simulink library "Library_SII_2018"  (R2018b)
settings: Solver=ode45  StartTime=0.0  StopTime=10.0  RelTol=1e-3  EnableMultiTasking=on
undefined symbols (not defined in the file or in its folder): coder, gcbh, r, simscape
libraries: fl_lib x157, nesl_utility x81, Library_SII2 x44, simulink x17, powerlib x12, mblibv1 x11, Simscape_SII_lib x11, elec_lib x10, Pneumatic_lib x4, $bdroot x2, peRmsMeasurement x1, powerlib_extras x1
(part 4 of 6)

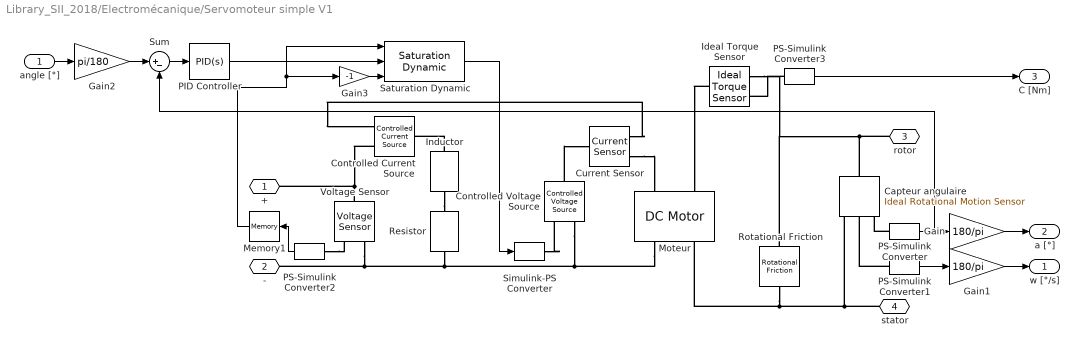
== system Library_SII_2018/Electromécanique/Servomoteur simple V1 ==
  angle [°] : Inport
  Capteur angulaire : fl_lib/Mechanical/Mechanical Sensors/Ideal Rotational Motion Sensor  offset=0 rad
  Controlled Current Source : fl_lib/Electrical/Electrical Sources/Controlled Current Source
  Controlled Voltage Source : fl_lib/Electrical/Electrical Sources/Controlled Voltage Source
  Current Sensor : fl_lib/Electrical/Electrical Sensors/Current Sensor
  Gain : Gain  Gain=180/pi
  Gain1 : Gain  Gain=180/pi
  Gain2 : Gain  Gain=pi/180
  Gain3 : Gain  Gain=-1
  Ideal Torque Sensor : fl_lib/Mechanical/Mechanical Sensors/Ideal Torque Sensor
  Inductor : fl_lib/Electrical/Electrical Elements/Inductor  l=L H  r=0 Ohm  g=1e-9 1/Ohm  i_specify=off  i_priority=High  i=0 A  i_nominal_specify=off  i_nominal_unit=A  i_nominal_value=1  v_specify=off  v_priority=High  v=0 V  v_nominal_specify=off  v_nominal_unit=V  v_nominal_value=1  i_L_specify=off  i_L_priority=High  i_L=0 A  i_L_nominal_specify=off  i_L_nominal_unit=A  i_L_nominal_value=1
  Memory1 : Memory  InheritSampleTime=on  LinearizeMemory=on
  Moteur : elec_lib/Actuators & Drivers/Rotational Actuators/DC Motor  parameterization=1  Ra=R Ohm  La=L H  emf_or_torque=1  Kv=K V/(rad/s)  Ki=6.876e-4 N*m/A  T_stall=2.4e-4 N*m  w_max=1.91e+4 rpm  w_rated=1.5e+4 rpm  P_rated=0.08 W  V_rated=1.5 V  J=0.001 kg*m^2  lam_param=1  lam=kv N*m/(rad/s)  i_noload=0 A  V_i_noload=1.5 V  speed0=0 rpm  alpha=0.00393 1/K  Tmeas=25 C  thermal_mass=100 J/K  initial_temperature=25 C
  PID Controller : simulink/Continuous/PID Controller  Controller=PID  Form=Parallel  TimeDomain=Continuous-time  SampleTime=-1  IntegratorMethod=Forward Euler  FilterMethod=Forward Euler  ControllerParametersSource=internal  P=P  I=I  D=D  UseFilter=on  N=100  TunerSelectOption=Transfer Function Based (PID Tuner App)  InitialConditionSource=internal  InitialConditionForIntegrator=0  InitialConditionForFilter=0  DifferentiatorICPrevScaledInput=0  ExternalReset=none  TrackingMode=off  Kt=1  LimitOutput=off  UpperSaturationLimit=inf  LowerSaturationLimit=-inf  LinearizeAsGain=on  AntiWindupMode=none  Kb=1  POutMin=[]  POutMax=[]  IOutMin=[]  IOutMax=[]  DOutMin=[]  DOutMax=[]  NOutMin=[]  NOutMax=[]  SumOutMin=[]  SumOutMax=[]  SaturationOutMin=[]  SaturationOutMax=[]  PParamMin=[]  PParamMax=[]  IParamMin=[]  IParamMax=[]  DParamMin=[]  DParamMax=[]  NParamMin=[]  NParamMax=[]  KbParamMin=[]  KbParamMax=[]  KtParamMin=[]  KtParamMax=[]  KbOutMin=[]  KbOutMax=[]  KtOutMin=[]  KtOutMax=[]  IntegratorOutMin=[]  IntegratorOutMax=[]  FilterOutMin=[]  FilterOutMax=[]  SumI1OutMin=[]  SumI1OutMax=[]  SumI2OutMin=[]  SumI2OutMax=[]  SumI3OutMin=[]  SumI3OutMax=[]  SumI4OutMin=[]  SumI4OutMax=[]  SumDOutMin=[]  SumDOutMax=[]  DifferentiatorOutMin=[]  DifferentiatorOutMax=[]  FilterDiffOutCoefMin=[]  FilterDiffOutCoefMax=[]  ReciprocalOutMin=[]  ReciprocalOutMax=[]  SumDenOutMin=[]  SumDenOutMax=[]  SumNumOutMin=[]  SumNumOutMax=[]  DivideOutMin=[]  DivideOutMax=[]  IntegratorContinuousStateAttributes=''  IntegratorStateMustResolveToSignalObject=off  IntegratorRTWStateStorageClass=Auto  FilterContinuousStateAttributes=''  FilterStateMustResolveToSignalObject=off  FilterRTWStateStorageClass=Auto  ParallelPVariant=InternalParameters  IdealPVariant=Disabled  IVariant=InternalParameters  DVariant=InternalParameters  IntegratorVariant=Continuous  SatVariant=Disabled  AWVariant=Passthrough  PCopyVariant=Disabled  TRVariant=Disabled  FdbkBlocksVariant=Forward  IdealPFdbkVariant=Disabled  SatFdbkVariant=Disabled  DerivativeFilterVariant=ContFilter  NVariant=InternalParameters  NCopyVariant=Disabled  FilterICVariant=InternalICsFilter  IntegratorICVariant=InternalICs  ExternalResetVariant=Disabled  TRSumVariant=Passthrough  SumFdbkVariant=Disabled  SumVariant=Sum_PID
  PS-Simulink Converter{,1..3} (4 alike) : nesl_utility/PS-Simulink Converter  PhysicalDomain=network_engine_domain  SubClassName=ps_output  LeftPortType=input  RightPortType=output  PseudoPeriodic=off  Frequencies=[]  Unit=1  AffineConversion=off
  Resistor : fl_lib/Electrical/Electrical Elements/Resistor  R=1/(1/R+1/R0) Ohm  i_specify=off  i_priority=High  i=0 A  i_nominal_specify=off  i_nominal_unit=A  i_nominal_value=1  v_specify=off  v_priority=High  v=0 V  v_nominal_specify=off  v_nominal_unit=V  v_nominal_value=1
  Rotational Friction : fl_lib/Mechanical/Rotational Elements/Rotational Friction  brkwy_trq=Cf*1.1 N*m  brkwy_vel=0.060623 rad/s  Col_trq=Cf N*m  visc_coef=0 N*m/(rad/s)  w_specify=off  w_priority=High  w=0 rad/s  w_nominal_specify=off  w_nominal_unit=rad/s  w_nominal_value=1  t_specify=off  t_priority=High  t=0 N*m  t_nominal_specify=off  t_nominal_unit=N*m  t_nominal_value=1
      settings: SourceProductName=Simscape
  Saturation Dynamic : simulink/Discontinuities/Saturation Dynamic  OutMin=[]  OutMax=[]  OutDataTypeStr=Inherit: Same as second input  OutDataType=fixdt(1, 16)  OutScaling=2^-10  DoSatur=off
  Simulink-PS Converter : nesl_utility/Simulink-PS Converter  PhysicalDomain=network_engine_domain  SubClassName=ps_input  LeftPortType=input  RightPortType=output  PseudoPeriodic=off  Frequencies=[]  NoiseDistribution=none  NoiseParameters=[]  Unit=1  AffineConversion=off  FilteringAndDerivatives=zero  SimscapeFilterOrder=1  InputFilterTimeConstant=0.001  UdotUserProvided=1
  Sum : Sum  Inputs=|+-
  Voltage Sensor : fl_lib/Electrical/Electrical Sensors/Voltage Sensor
  + : PMIOPort  Side=Left
  - : PMIOPort  Port=2  Side=Left
  rotor : PMIOPort  Port=3  Side=Right
  stator : PMIOPort  Port=4  Side=Right
  w [°/s] : Outport
  a [°] : Outport  Port=2
  C [Nm] : Outport  Port=3
  wires:
  PS-Simulink Converter3/1 -> C [Nm]/1
  PS-Simulink Converter1/1 -> Gain1/1
  Sum/1 -> PID Controller/1
  angle [°]/1 -> Gain2/1
  Gain/1 -> a [°]/1
  Gain1/1 -> w [°/s]/1
  Gain2/1 -> Sum/1
  PID Controller/1 -> Saturation Dynamic/2
  Saturation Dynamic/1 -> Simulink-PS Converter/1
  Gain3/1 -> Saturation Dynamic/3
  Memory1/1 -> Saturation Dynamic/1, Gain3/1
  PS-Simulink Converter/1 -> Sum/2, Gain/1
  PS-Simulink Converter2/1 -> Memory1/1
  connections:
  PS-Simulink Converter3/LConn1 -- Ideal Torque Sensor/RConn2
  Ideal Torque Sensor/LConn1 -- Moteur/LConn2
  stator/RConn1 -- Rotational Friction/RConn1 -- Moteur/RConn2 -- Capteur angulaire/RConn1
  PS-Simulink Converter1/LConn1 -- Capteur angulaire/RConn2
  PS-Simulink Converter/LConn1 -- Capteur angulaire/RConn3
  Capteur angulaire/LConn1 -- Rotational Friction/LConn1 -- Ideal Torque Sensor/RConn1 -- rotor/RConn1
  Moteur/RConn1 -- Controlled Voltage Source/RConn2 -- Resistor/RConn1 -- -/RConn1 -- Voltage Sensor/RConn2
  Controlled Voltage Source/LConn1 -- Current Sensor/LConn1
  Controlled Current Source/RConn2 -- Voltage Sensor/LConn1 -- +/RConn1
  Simulink-PS Converter/RConn1 -- Controlled Voltage Source/RConn1
  Current Sensor/RConn2 -- Moteur/LConn1
  Current Sensor/RConn1 -- Controlled Current Source/RConn1
  PS-Simulink Converter2/LConn1 -- Voltage Sensor/RConn1
  Inductor/LConn1 -- Controlled Current Source/LConn1
  Inductor/RConn1 -- Resistor/LConn1

== system Library_SII_2018/Electronique/Ampèremètre ==
  Current Sensor : fl_lib/Electrical/Electrical Sensors/Current Sensor
  S-PS : nesl_utility/PS-Simulink Converter  PhysicalDomain=network_engine_domain  SubClassName=ps_output  LeftPortType=input  RightPortType=output  PseudoPeriodic=off  Frequencies=[]  Unit=A  AffineConversion=off
  Conn1 : PMIOPort  Side=Left
  Conn2 : PMIOPort  Port=2  Side=Right
  Out1 : Outport
  wires:
  S-PS/1 -> Out1/1
  connections:
  Current Sensor/RConn1 -- S-PS/LConn1
  Conn2/RConn1 -- Current Sensor/RConn2
  Conn1/RConn1 -- Current Sensor/LConn1

== system Library_SII_2018/Electronique/Bobine entrée ==
  Electromagnetic Converter : fl_lib/Magnetic/Magnetic Elements/Electromagnetic Converter  Nw=N  i_specify=off  i_priority=None  i=0 A  i_nominal_specify=off  i_nominal_unit=A  i_nominal_value=1  v_specify=off  v_priority=None  v=0 V  v_nominal_specify=off  v_nominal_unit=V  v_nominal_value=1  mmf_specify=off  mmf_priority=None  mmf=0 A  mmf_nominal_specify=off  mmf_nominal_unit=A  mmf_nominal_value=1  phi_specify=off  phi_priority=High  phi=0 Wb  phi_nominal_specify=off  phi_nominal_unit=Wb  phi_nominal_value=1
      settings: SourceProductName=Simscape  SourceProductBaseCode=SS
  Fundamental Reluctance : fl_lib/Magnetic/Magnetic Elements/Fundamental Reluctance  R=4*l/(mu0*pi*D^2) 1/H  phi_specify=off  phi_priority=None  phi=0 Wb  phi_nominal_specify=off  phi_nominal_unit=Wb  phi_nominal_value=1  mmf_specify=off  mmf_priority=None  mmf=0 A  mmf_nominal_specify=off  mmf_nominal_unit=A  mmf_nominal_value=1
      settings: SourceProductName=Simscape  SourceProductBaseCode=SS
  Inductor : fl_lib/Electrical/Electrical Elements/Inductor  l=mu0*pi*D^2/4*N^2/l H  r=0 Ohm  g=1e-20 1/Ohm  i_specify=off  i_priority=None  i=0 A  i_nominal_specify=off  i_nominal_unit=A  i_nominal_value=1  v_specify=off  v_priority=None  v=0 V  v_nominal_specify=off  v_nominal_unit=V  v_nominal_value=1  i_L_specify=off  i_L_priority=High  i_L=0 A  i_L_nominal_specify=off  i_L_nominal_unit=A  i_L_nominal_value=1
  Resistor : fl_lib/Electrical/Electrical Elements/Resistor  R=rho*pi*D*N/s Ohm  i_specify=off  i_priority=None  i=0 A  i_nominal_specify=off  i_nominal_unit=A  i_nominal_value=1  v_specify=off  v_priority=None  v=0 V  v_nominal_specify=off  v_nominal_unit=V  v_nominal_value=1
  + : PMIOPort  Side=Left
  - : PMIOPort  Port=2  Side=Left
  N : PMIOPort  Port=3  Side=Right
  S : PMIOPort  Port=4  Side=Right
  connections:
  -/RConn1 -- Inductor/LConn1
  +/RConn1 -- Resistor/LConn1
  Inductor/RConn1 -- Electromagnetic Converter/LConn2
  Fundamental Reluctance/RConn1 -- S/RConn1 -- Electromagnetic Converter/RConn2
  Resistor/RConn1 -- Electromagnetic Converter/LConn1
  Electromagnetic Converter/RConn1 -- Fundamental Reluctance/LConn1 -- N/RConn1

== system Library_SII_2018/Electronique/Cellule Photovoltaique SPS ==
  Ta : Inport
  Ir : Inport  Port=2
  Add : Sum  Inputs=-+
  Courant de saturation diode : Subsystem
  Courant diode : Subsystem
  Courant gégéré par l'éclairement : Subsystem
  Estimation température cellule : Subsystem
  Fcn : Fcn  Expr=u(1)+beta*(u(2)-Tjref)
  Is : powerlib/Electrical Sources/Controlled Current Source  Initialize=on  Source_Type=AC  Amplitude=0  Phase=0  Frequency=0  Measurements=None
      settings: SourceProductName=Simscape Electrical
  Mux : Mux  Inputs=2
  Rs : powerlib/Elements/Series RLC Branch  LConnTagsString=__new0  RConnTagsString=__new0  BranchType=R  Resistance=Rs  Inductance=1e-3  SetiL0=off  InitialCurrent=0  Capacitance=1e-6  Setx0=off  InitialVoltage=0  Measurements=None
      settings: SourceProductName=Simscape Electrical
  Rsh : powerlib/Elements/Series RLC Branch  LConnTagsString=__new0  RConnTagsString=__new0  BranchType=R  Resistance=Rsh  Inductance=1e-3  SetiL0=off  InitialCurrent=0  Capacitance=1e-6  Setx0=off  InitialVoltage=0  Measurements=None
      settings: SourceProductName=Simscape Electrical
  Température optimale (constructeur) : Constant  Value=45
  Tension thermique : Subsystem
  Transport Delay : TransportDelay  DelayTime=0.001
  V : powerlib/Measurements/Voltage Measurement  PhasorSimulation=off  OutputType=Complex  PSBequivalent=0
      settings: SourceProductName=Simscape Electrical
  + : PMIOPort  Tag=PMCPort  Side=Right
  - : PMIOPort  Tag=PMCPort  Port=2  Side=Right
  wires:
  Add/1 -> Is/1
  Estimation température cellule/1(Tj) -> Courant gégéré par l'éclairement/1(Tj), Tension thermique/1(Tj (°C)), Courant de saturation diode/1(Tj)
  Température optimale (constructeur)/1 -> Estimation température cellule/1(noct)
  Ta/1 -> Estimation température cellule/2(Ta)
  Ir/1 -> Estimation température cellule/3(Ir), Courant gégéré par l'éclairement/2(Ir)
  Courant gégéré par l'éclairement/1(Iph) -> Add/2
  Courant diode/1(Id) -> Add/1
  Mux/1 -> Fcn/1
  V/1 -> Courant diode/1(Vd)
  Tension thermique/1(Vt (V)) -> Courant diode/3(Vt), Courant de saturation diode/2(Vt)
  Courant de saturation diode/1(Id0) -> Courant diode/2(I0d)
  connections:
  V/LConn2 -- -/RConn1 -- Is/LConn1 -- Rsh/RConn1
  Is/RConn1 -- Rs/LConn1 -- V/LConn1 -- Rsh/LConn1
  Rs/RConn1 -- +/RConn1

== system Library_SII_2018/Electronique/Cellule Photovoltaique avec capteurs U et I SimElectronics ==
  Ir : Inport
  Constant : Constant  Value=shunt
  Current Sensor : fl_lib/Electrical/Electrical Sensors/Current Sensor
  PS-Simulink Converter : nesl_utility/PS-Simulink Converter  PhysicalDomain=network_engine_domain  SubClassName=ps_output  LeftPortType=input  RightPortType=output  PseudoPeriodic=off  Frequencies=[]  Unit=1  AffineConversion=off
  PS-Simulink Converter1 : nesl_utility/PS-Simulink Converter  PhysicalDomain=network_engine_domain  SubClassName=ps_output  LeftPortType=input  RightPortType=output  PseudoPeriodic=off  Frequencies=[]  Unit=1  AffineConversion=off
  Simulink-PS Converter : nesl_utility/Simulink-PS Converter  PhysicalDomain=network_engine_domain  SubClassName=ps_input  LeftPortType=input  RightPortType=output  PseudoPeriodic=off  Frequencies=[]  NoiseDistribution=none  NoiseParameters=[]  Unit=1  AffineConversion=off  FilteringAndDerivatives=zero  SimscapeFilterOrder=1  InputFilterTimeConstant=.001  UdotUserProvided=0
  Simulink-PS Converter1 : nesl_utility/Simulink-PS Converter  PhysicalDomain=network_engine_domain  SubClassName=ps_input  LeftPortType=input  RightPortType=output  PseudoPeriodic=off  Frequencies=[]  NoiseDistribution=none  NoiseParameters=[]  Unit=1  AffineConversion=off  FilteringAndDerivatives=zero  SimscapeFilterOrder=1  InputFilterTimeConstant=.001  UdotUserProvided=0
  Solar Cell : elec_lib/Sources/Solar Cell  prm=1  Isc=Icc A  Voc=Vco V  Is=1e-6 A  Is2=0 A  Iph=7.34 A  Ir0=IRef W/m^2  ec=Qf  N2=2  Rs=0 Ohm  Rp=Inf Ohm  N_series=1  TIPH1=0 1/K  EG=1.11 eV  TXIS1=3  TXIS2=3  TRS1=0  TRP1=0  Tmeas=TRef C  TFIXED=Tcell C  thermal_mass=100 J/K  initial_temperature=25 C
      settings: SourceProductName=Simscape Electronics  SourceProductBaseCode=SN
  Switch : fl_lib/Electrical/Electrical Elements/Switch  R_closed=1e-8 Ohm  G_open=1e-8 1/Ohm  Threshold=0  i_specify=off  i_priority=High  i=0 A  i_nominal_specify=off  i_nominal_unit=A  i_nominal_value=1  v_specify=off  v_priority=High  v=0 V  v_nominal_specify=off  v_nominal_unit=V  v_nominal_value=1
      settings: SourceProductName=Simscape
  Voltage Sensor : fl_lib/Electrical/Electrical Sensors/Voltage Sensor
  + : PMIOPort  Side=Right
  - : PMIOPort  Port=2  Side=Right
  I : Outport
  U : Outport  Port=2
  wires:
  Ir/1 -> Simulink-PS Converter1/1
  PS-Simulink Converter/1 -> I/1
  PS-Simulink Converter1/1 -> U/1
  Constant/1 -> Simulink-PS Converter/1
  connections:
  Simulink-PS Converter1/RConn1 -- Solar Cell/LConn1
  Switch/RConn2 -- Voltage Sensor/RConn2 -- -/RConn1 -- Solar Cell/RConn1
  Voltage Sensor/LConn1 -- Current Sensor/RConn2 -- +/RConn1
  Voltage Sensor/RConn1 -- PS-Simulink Converter1/LConn1
  Current Sensor/RConn1 -- PS-Simulink Converter/LConn1
  Switch/LConn1 -- Current Sensor/LConn1 -- Solar Cell/LConn2
  Simulink-PS Converter/RConn1 -- Switch/RConn1

== system Library_SII_2018/Electronique/Diode ==
  Tj (°C) : Inport
  Courant de saturation diode : Subsystem
  Courant diode : Subsystem
  Is : powerlib/Electrical Sources/Controlled Current Source  Initialize=on  Source_Type=AC  Amplitude=0  Phase=0  Frequency=0  Measurements=None
      settings: SourceProductName=Simscape Electrical
  Tension thermique : Subsystem
  V : powerlib/Measurements/Voltage Measurement  PhasorSimulation=off  OutputType=Complex  PSBequivalent=0
      settings: SourceProductName=Simscape Electrical
  C : PMIOPort  Tag=PMCPort  Side=Right
  A : PMIOPort  Tag=PMCPort  Port=2  Side=Left
  wires:
  Courant diode/1(Id) -> Is/1
  V/1 -> Courant diode/1(Vd)
  Courant de saturation diode/1(Id0) -> Courant diode/2(I0d)
  Tj (°C)/1 -> Courant de saturation diode/1(Tj), Tension thermique/1(Tj (°C))
  Tension thermique/1(Vt) -> Courant diode/3(Vt)
  connections:
  Is/LConn1 -- C/RConn1 -- V/LConn2
  Is/RConn1 -- A/RConn1 -- V/LConn1

== system Library_SII_2018/Electronique/Hacheur (PWM) ==
  Consigne (0 --> 100) : Inport
  Controlled Voltage Source1 : fl_lib/Electrical/Electrical Sources/Controlled Voltage Source
  Gain1 : Gain  Gain=A  OutDataTypeStr=double
  Relational Operator : RelationalOperator  RndMeth=Nearest
  Repeating Sequence : simulink/Sources/Repeating Sequence  rep_seq_t=[0 1/f]  rep_seq_y=[0 100]
  Simulink-PS Converter : nesl_utility/Simulink-PS Converter  PhysicalDomain=network_engine_domain  SubClassName=ps_input  LeftPortType=input  RightPortType=output  PseudoPeriodic=off  Frequencies=[]  NoiseDistribution=none  NoiseParameters=[]  Unit=1  AffineConversion=off  FilteringAndDerivatives=zero  SimscapeFilterOrder=1  InputFilterTimeConstant=0.001  UdotUserProvided=1
  + : PMIOPort  Side=Right
  - : PMIOPort  Port=2  Side=Right
  Tension : Outport
  wires:
  Relational Operator/1 -> Gain1/1
  Gain1/1 -> Tension/1, Simulink-PS Converter/1
  Consigne (0 --> 100)/1 -> Relational Operator/1
  Repeating Sequence/1 -> Relational Operator/2
  connections:
  Controlled Voltage Source1/RConn1 -- Simulink-PS Converter/RConn1
  -/RConn1 -- Controlled Voltage Source1/RConn2
  +/RConn1 -- Controlled Voltage Source1/LConn1

== system Library_SII_2018/Electronique/Hacheur (PWM) Tension variable ==
  Consigne (0 --> 100) : Inport
  Tension [V] : Inport  Port=2
  Controlled Voltage Source1 : fl_lib/Electrical/Electrical Sources/Controlled Voltage Source
  Product : Product
  Relational Operator : RelationalOperator  RndMeth=Nearest
  Repeating Sequence : simulink/Sources/Repeating Sequence  rep_seq_t=[0 1/f]  rep_seq_y=[0 100]
  Simulink-PS Converter : nesl_utility/Simulink-PS Converter  PhysicalDomain=network_engine_domain  SubClassName=ps_input  LeftPortType=input  RightPortType=output  PseudoPeriodic=off  Frequencies=[]  NoiseDistribution=none  NoiseParameters=[]  Unit=1  AffineConversion=off  FilteringAndDerivatives=zero  SimscapeFilterOrder=1  InputFilterTimeConstant=0.001  UdotUserProvided=1
  + : PMIOPort  Side=Right
  - : PMIOPort  Port=2  Side=Right
  Tension : Outport
  wires:
  Repeating Sequence/1 -> Relational Operator/2
  Consigne (0 --> 100)/1 -> Relational Operator/1
  Product/1 -> Simulink-PS Converter/1, Tension/1
  Relational Operator/1 -> Product/2
  Tension [V]/1 -> Product/1
  connections:
  +/RConn1 -- Controlled Voltage Source1/LConn1
  -/RConn1 -- Controlled Voltage Source1/RConn2
  Controlled Voltage Source1/RConn1 -- Simulink-PS Converter/RConn1

== system Library_SII_2018/Electronique/Interrupteur ==
  In1 : Inport
  S-PS1 : nesl_utility/Simulink-PS Converter  PhysicalDomain=network_engine_domain  SubClassName=ps_input  LeftPortType=input  RightPortType=output  PseudoPeriodic=off  Frequencies=[]  NoiseDistribution=none  NoiseParameters=[]  Unit=1  AffineConversion=off  FilteringAndDerivatives=zero  SimscapeFilterOrder=1  InputFilterTimeConstant=.001  UdotUserProvided=0
  Switch : fl_lib/Electrical/Electrical Elements/Switch  R_closed=1e-8 Ohm  G_open=1e-8 1/Ohm  Threshold=0  i_specify=off  i_priority=High  i=0 A  i_nominal_specify=off  i_nominal_unit=A  i_nominal_value=1  v_specify=off  v_priority=High  v=0 V  v_nominal_specify=off  v_nominal_unit=V  v_nominal_value=1
      settings: SourceProductName=Simscape
  Conn1 : PMIOPort  Side=Left
  Conn2 : PMIOPort  Port=2  Side=Right
  wires:
  In1/1 -> S-PS1/1
  connections:
  S-PS1/RConn1 -- Switch/RConn1
  Conn1/RConn1 -- Switch/LConn1
  Conn2/RConn1 -- Switch/RConn2

== system Library_SII_2018/Electronique/Mesure Puissance RMS ==
  Amperemetre : $bdroot/Electronique/Ampèremètre
  Mux : Mux  Inputs=3
  Product : Product
  RMS Measurement : peRmsMeasurement/RMS Measurement  LabelModeActiveChoice=Total  F=ff  SpecifyHarmonics=off  K=[0 1 2]  Ts=0
  Voltmetre : $bdroot/Electronique/Voltmètre
  E : PMIOPort  Side=Left
  Ref : PMIOPort  Port=2  Side=Left
  S : PMIOPort  Port=3  Side=Right
  "[I, U, P]" : Outport
  wires:
  Mux/1 -> RMS Measurement/1
  RMS Measurement/1 -> "[I, U, P]"/1
  Product/1 -> Mux/3  "Puissance"
  Voltmetre/1 -> Product/2, Mux/2  "Upv"
  Amperemetre/1 -> Product/1, Mux/1  "Ipv"
  connections:
  Amperemetre/RConn1 -- S/RConn1 -- Voltmetre/LConn1
  Voltmetre/RConn1 -- Ref/RConn1
  Amperemetre/LConn1 -- E/RConn1

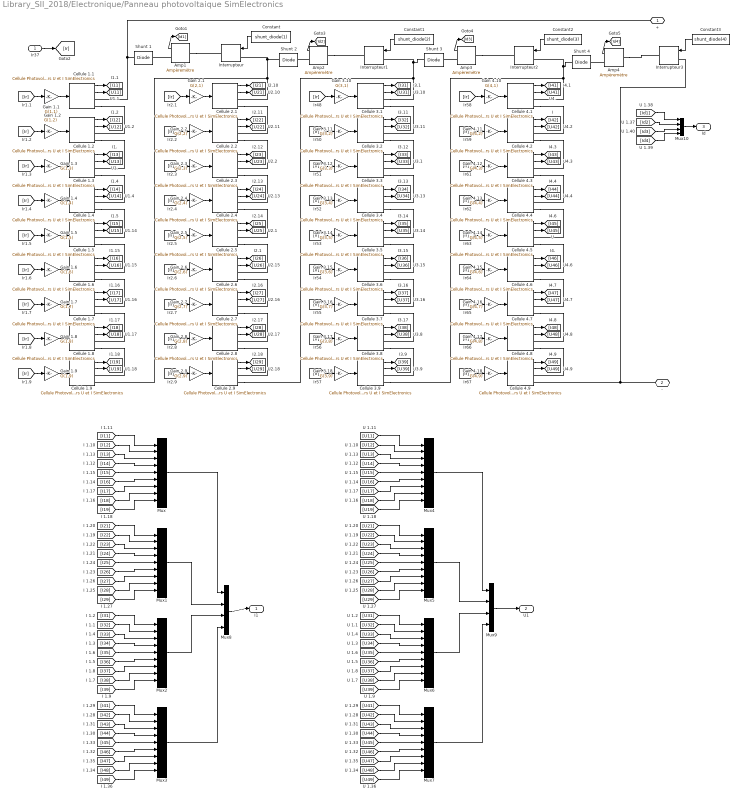
== system Library_SII_2018/Electronique/Panneau photovoltaique SimElectronics ==
  Ir37 : Inport
  Amp{1..4} (4 alike) : Library_SII2/Electronique/Ampèremètre
  Cellule 1.1 : Library_SII2/Electronique/Cellule Photovoltaique avec capteurs U et I SimElectronics  typcell=polycristallin  Icc=Icc  Vco=Vco  Tcell=Tcell  shunt=0  mesure=off  IRef=1000  TRef=25  Qf=1.4
  Cellule 1.{2..8} (7 alike) : Library_SII2/Electronique/Cellule Photovoltaique avec capteurs U et I SimElectronics  typcell=polycristallin  Icc=Icc  Vco=Vco  Tcell=Tcell  shunt=0  mesure=off  IRef=1000  TRef=25  Qf=1.5
  Cellule 1.9 : Library_SII2/Electronique/Cellule Photovoltaique avec capteurs U et I SimElectronics  typcell=polycristallin  Icc=Icc  Vco=Vco  Tcell=Tcell  shunt=1  mesure=off  IRef=1000  TRef=25  Qf=1.5
  Cellule 2.{1..7} (7 alike) : Library_SII2/Electronique/Cellule Photovoltaique avec capteurs U et I SimElectronics  typcell=polycristallin  Icc=Icc  Vco=Vco  Tcell=Tcell  shunt=0  mesure=off  IRef=1000  TRef=25  Qf=1.5
  Cellule 2.8 : Library_SII2/Electronique/Cellule Photovoltaique avec capteurs U et I SimElectronics  typcell=polycristallin  Icc=Icc  Vco=Vco  Tcell=Tcell  shunt=0  mesure=off  IRef=1000  TRef=25  Qf=10
  Cellule 2.9 : Library_SII2/Electronique/Cellule Photovoltaique avec capteurs U et I SimElectronics  typcell=polycristallin  Icc=Icc  Vco=Vco  Tcell=Tcell  shunt=1  mesure=off  IRef=1000  TRef=25  Qf=1.5
  Cellule 3.{1..8} (8 alike) : Library_SII2/Electronique/Cellule Photovoltaique avec capteurs U et I SimElectronics  typcell=polycristallin  Icc=Icc  Vco=Vco  Tcell=Tcell  shunt=0  mesure=off  IRef=1000  TRef=25  Qf=1.5
  Cellule 3.9 : Library_SII2/Electronique/Cellule Photovoltaique avec capteurs U et I SimElectronics  typcell=polycristallin  Icc=Icc  Vco=Vco  Tcell=Tcell  shunt=1  mesure=off  IRef=1000  TRef=25  Qf=1.5
  Cellule 4.{1..8} (8 alike) : Library_SII2/Electronique/Cellule Photovoltaique avec capteurs U et I SimElectronics  typcell=polycristallin  Icc=Icc  Vco=Vco  Tcell=Tcell  shunt=0  mesure=off  IRef=1000  TRef=25  Qf=1.5
  Cellule 4.9 : Library_SII2/Electronique/Cellule Photovoltaique avec capteurs U et I SimElectronics  typcell=polycristallin  Icc=Icc  Vco=Vco  Tcell=Tcell  shunt=1  mesure=off  IRef=1000  TRef=25  Qf=1.5
  Constant : Constant  Value=shunt_diode(1)
  Constant1 : Constant  Value=shunt_diode(2)
  Constant2 : Constant  Value=shunt_diode(3)
  Constant3 : Constant  Value=shunt_diode(4)
  Gain 1.1 : Gain  Gain=G(1,1)
  Gain 1.2 : Gain  Gain=G(1,2)
  Gain 1.3 : Gain  Gain=G(1,3)
  Gain 1.4 : Gain  Gain=G(1,4)
  Gain 1.5 : Gain  Gain=G(1,5)
  Gain 1.6 : Gain  Gain=G(1,6)
  Gain 1.7 : Gain  Gain=G(1,7)
  Gain 1.8 : Gain  Gain=G(1,8)
  Gain 1.9 : Gain  Gain=G(1,9)
  Gain 2.1 : Gain  Gain=G(2,1)
  Gain 2.2 : Gain  Gain=G(2,2)
  Gain 2.3 : Gain  Gain=G(2,3)
  Gain 2.4 : Gain  Gain=G(2,4)
  Gain 2.5 : Gain  Gain=G(2,5)
  Gain 2.6 : Gain  Gain=G(2,6)
  Gain 2.7 : Gain  Gain=G(2,7)
  Gain 2.8 : Gain  Gain=G(2,8)
  Gain 2.9 : Gain  Gain=G(2,9)
  Gain 3.10 : Gain  Gain=G(3,1)
  Gain 3.11 : Gain  Gain=G(3,2)
  Gain 3.12 : Gain  Gain=G(3,3)
  Gain 3.13 : Gain  Gain=G(3,4)
  Gain 3.14 : Gain  Gain=G(3,5)
  Gain 3.15 : Gain  Gain=G(3,6)
  Gain 3.16 : Gain  Gain=G(3,7)
  Gain 3.17 : Gain  Gain=G(3,8)
  Gain 3.18 : Gain  Gain=G(3,9)
  Gain 4.10 : Gain  Gain=G(4,1)
  Gain 4.11 : Gain  Gain=G(4,2)
  Gain 4.12 : Gain  Gain=G(4,3)
  Gain 4.13 : Gain  Gain=G(4,4)
  Gain 4.14 : Gain  Gain=G(4,5)
  Gain 4.15 : Gain  Gain=G(4,6)
  Gain 4.16 : Gain  Gain=G(4,7)
  Gain 4.17 : Gain  Gain=G(4,8)
  Gain 4.18 : Gain  Gain=G(4,9)
  Interrupteur{,1..3} (4 alike) : Library_SII2/Electronique/Interrupteur
  Mux{,1..7} (8 alike) : Mux  Inputs=9
  Mux10 : Mux
  Mux8 : Mux
  Mux9 : Mux
  Shunt {1..4} (4 alike) : elec_lib/Semiconductor Devices/Diode  ModelType=1  Vf=0.6 V  Ron=0.3 Ohm  Goff=1e-8 S  Rz=0.3 Ohm  Vz=50 V  C_PWL=5 pF  prmExp=1  I12=[ 0.0137 0.545 ] A  V12=[ 0.6 0.7 ] V  I1=0.0137 A  V1=0.6 V  IS=1e-12 A  ec=1  RS=0.01 Ohm  Tmeas=25 C  BV=Inf V  C_param=1  CJ0=5 pF  VJ=1 V  Mgrad=0.5  Vvec=[ 0.1 10 100 ] V  Cvec=[ 3.5 1 0.4 ] pF  FC=0.5  Q_param=1  Irrm=-7.15 A  iF=4 A  didt=-750 A/us  trr=115 ns  TT=50 ns  tau=100 ns  T_param=1  IS_T2=1.25e-7 A  I1_T2=0.245 A  V1_T2=0.5 V  Tmeas2=125 C  EG_param=1  EG=1.11 eV  XTI_param=1  XTI=3  dBVdT=0 V/K  Tdevice=25 C  i_capacitor_specify=off  i_capacitor_priority=High  i_capacitor=0 A  i_capacitor_nominal_specify=off  i_capacitor_nominal_unit=A  i_capacitor_nominal_value=1  v_capacitor_specify=off  v_capacitor_priority=None  v_capacitor=0 V  v_capacitor_nominal_specify=off  v_capacitor_nominal_unit=V  v_capacitor_nominal_value=1  Rth=[ 0 10 ] K/W  thermal_mass_parameterization=1  thermal_mass=[ 0 1 ] J/K  thermal_time_constant=[ 0 10 ] s  thermal_mass_initial_temperatures=[ 25 25 ] C
      settings: SourceProductName=Simscape Electronics  SourceProductBaseCode=SN
  + : PMIOPort  Side=Right
  - : PMIOPort  Port=2  Side=Right
  I1 : Outport
  U1 : Outport  Port=2
  Id : Outport  Port=3
  wires:
  Ir37/1 -> [Ir]
  [Ir] -> Gain 1.1/1
  Gain 1.1/1 -> Cellule 1.1/1
  Cellule 1.1/1 -> [I11]
  Cellule 1.1/2 -> [U11]
  [Ir] -> Gain 1.2/1
  Gain 1.2/1 -> Cellule 1.2/1
  Cellule 1.2/1 -> [I12]
  Cellule 1.2/2 -> [U12]
  [Ir] -> Gain 1.3/1
  Gain 1.3/1 -> Cellule 1.3/1
  Cellule 1.3/1 -> [I13]
  Cellule 1.3/2 -> [U13]
  [Ir] -> Gain 1.4/1
  Gain 1.4/1 -> Cellule 1.4/1
  Cellule 1.4/1 -> [I14]
  Cellule 1.4/2 -> [U14]
  [Ir] -> Gain 1.5/1
  Gain 1.5/1 -> Cellule 1.5/1
  Cellule 1.5/1 -> [I15]
  Cellule 1.5/2 -> [U15]
  [Ir] -> Gain 1.6/1
  Gain 1.6/1 -> Cellule 1.6/1
  Cellule 1.6/1 -> [I16]
  Cellule 1.6/2 -> [U16]
  [Ir] -> Gain 1.7/1
  Gain 1.7/1 -> Cellule 1.7/1
  Cellule 1.7/1 -> [I17]
  Cellule 1.7/2 -> [U17]
  [Ir] -> Gain 1.8/1
  Gain 1.8/1 -> Cellule 1.8/1
  Cellule 1.8/1 -> [I18]
  Cellule 1.8/2 -> [U18]
  [Ir] -> Gain 1.9/1
  Gain 1.9/1 -> Cellule 1.9/1
  Cellule 1.9/1 -> [I19]
  Cellule 1.9/2 -> [U19]
  [Ir] -> Gain 2.1/1
  Gain 2.1/1 -> Cellule 2.1/1
  Cellule 2.1/1 -> [I21]
  Cellule 2.1/2 -> [U21]
  [Ir] -> Gain 2.2/1
  Gain 2.2/1 -> Cellule 2.2/1
  Cellule 2.2/1 -> [I22]
  Cellule 2.2/2 -> [U22]
  [Ir] -> Gain 2.3/1
  Gain 2.3/1 -> Cellule 2.3/1
  Cellule 2.3/1 -> [I23]
  Cellule 2.3/2 -> [U23]
  [Ir] -> Gain 2.4/1
  Gain 2.4/1 -> Cellule 2.4/1
  Cellule 2.4/1 -> [I24]
  Cellule 2.4/2 -> [U24]
  [Ir] -> Gain 2.5/1
  Gain 2.5/1 -> Cellule 2.5/1
  Cellule 2.5/1 -> [I25]
  Cellule 2.5/2 -> [U25]
  [Ir] -> Gain 2.6/1
  Gain 2.6/1 -> Cellule 2.6/1
  Cellule 2.6/1 -> [I26]
  Cellule 2.6/2 -> [U26]
  [Ir] -> Gain 2.7/1
  Gain 2.7/1 -> Cellule 2.7/1
  Cellule 2.7/1 -> [I27]
  Cellule 2.7/2 -> [U27]
  [Ir] -> Gain 2.8/1
  Gain 2.8/1 -> Cellule 2.8/1
  Cellule 2.8/1 -> [I28]
  Cellule 2.8/2 -> [U28]
  [Ir] -> Gain 2.9/1
  Gain 2.9/1 -> Cellule 2.9/1
  Cellule 2.9/1 -> [I29]
  Cellule 2.9/2 -> [U29]
  [Ir] -> Gain 3.10/1
  Gain 3.10/1 -> Cellule 3.1/1
  Cellule 3.1/1 -> [I31]
  Cellule 3.1/2 -> [U31]
  [Ir] -> Gain 3.11/1
  Gain 3.11/1 -> Cellule 3.2/1
  Cellule 3.2/1 -> [I32]
  Cellule 3.2/2 -> [U32]
  [Ir] -> Gain 3.12/1
  Gain 3.12/1 -> Cellule 3.3/1
  Cellule 3.3/1 -> [I33]
  Cellule 3.3/2 -> [U33]
  [Ir] -> Gain 3.13/1
  Gain 3.13/1 -> Cellule 3.4/1
  Cellule 3.4/1 -> [I34]
  Cellule 3.4/2 -> [U34]
  [Ir] -> Gain 3.14/1
  Gain 3.14/1 -> Cellule 3.5/1
  Cellule 3.5/1 -> [I35]
  Cellule 3.5/2 -> [U35]
  [Ir] -> Gain 3.15/1
  Gain 3.15/1 -> Cellule 3.6/1
  Cellule 3.6/1 -> [I36]
  Cellule 3.6/2 -> [U36]
  [Ir] -> Gain 3.16/1
  Gain 3.16/1 -> Cellule 3.7/1
  Cellule 3.7/1 -> [I37]
  Cellule 3.7/2 -> [U37]
  [Ir] -> Gain 3.17/1
  Gain 3.17/1 -> Cellule 3.8/1
  Cellule 3.8/1 -> [I38]
  Cellule 3.8/2 -> [U38]
  [Ir] -> Gain 3.18/1
  Gain 3.18/1 -> Cellule 3.9/1
  Cellule 3.9/1 -> [I39]
  Cellule 3.9/2 -> [U39]
  [Ir] -> Gain 4.10/1
  Gain 4.10/1 -> Cellule 4.1/1
  Cellule 4.1/1 -> [I41]
  Cellule 4.1/2 -> [U41]
  [Ir] -> Gain 4.11/1
  Gain 4.11/1 -> Cellule 4.2/1
  Cellule 4.2/1 -> [I42]
  Cellule 4.2/2 -> [U42]
  [Ir] -> Gain 4.12/1
  Gain 4.12/1 -> Cellule 4.3/1
  Cellule 4.3/1 -> [I43]
  Cellule 4.3/2 -> [U43]
  [Ir] -> Gain 4.13/1
  Gain 4.13/1 -> Cellule 4.4/1
  Cellule 4.4/1 -> [I44]
  Cellule 4.4/2 -> [U44]
  [Ir] -> Gain 4.14/1
  Gain 4.14/1 -> Cellule 4.5/1
  Cellule 4.5/1 -> [I45]
  Cellule 4.5/2 -> [U45]
  [Ir] -> Gain 4.15/1
  Gain 4.15/1 -> Cellule 4.6/1
  Cellule 4.6/1 -> [I46]
  Cellule 4.6/2 -> [U46]
  [Ir] -> Gain 4.16/1
  Gain 4.16/1 -> Cellule 4.7/1
  Cellule 4.7/1 -> [I47]
  Cellule 4.7/2 -> [U47]
  [Ir] -> Gain 4.17/1
  Gain 4.17/1 -> Cellule 4.8/1
  Cellule 4.8/1 -> [I48]
  Cellule 4.8/2 -> [U48]
  [Ir] -> Gain 4.18/1
  Gain 4.18/1 -> Cellule 4.9/1
  Cellule 4.9/1 -> [I49]
  Cellule 4.9/2 -> [U49]
  [I11] -> Mux/1
  [I12] -> Mux/2
  [I13] -> Mux/3
  [I14] -> Mux/4
  [I15] -> Mux/5
  [I19] -> Mux/9
  [I18] -> Mux/8
  [I17] -> Mux/7
  [I16] -> Mux/6
  [I25] -> Mux1/5
  [I21] -> Mux1/1
  [I22] -> Mux1/2
  [I23] -> Mux1/3
  [I24] -> Mux1/4
  [I26] -> Mux1/6
  [I29] -> Mux1/9
  [I28] -> Mux1/8
  [I27] -> Mux1/7
  [I35] -> Mux2/5
  [I45] -> Mux3/5
  [U15] -> Mux4/5
  [U25] -> Mux5/5
  [U35] -> Mux6/5
  [U45] -> Mux7/5
  Mux1/1 -> Mux8/2
  Mux/1 -> Mux8/1
  Mux2/1 -> Mux8/3
  Mux3/1 -> Mux8/4
  Mux5/1 -> Mux9/2
  Mux4/1 -> Mux9/1
  Mux6/1 -> Mux9/3
  Mux7/1 -> Mux9/4
  [I31] -> Mux2/1
  [I39] -> Mux2/9
  [I38] -> Mux2/8
  [I37] -> Mux2/7
  [I36] -> Mux2/6
  [I32] -> Mux2/2
  [I33] -> Mux2/3
  [I34] -> Mux2/4
  [I41] -> Mux3/1
  [I42] -> Mux3/2
  [I43] -> Mux3/3
  [I49] -> Mux3/9
  [I48] -> Mux3/8
  [I47] -> Mux3/7
  [I46] -> Mux3/6
  [I44] -> Mux3/4
  [U11] -> Mux4/1
  [U19] -> Mux4/9
  [U21] -> Mux5/1
  [U29] -> Mux5/9
  [U31] -> Mux6/1
  [U39] -> Mux6/9
  [U41] -> Mux7/1
  [U49] -> Mux7/9
  [U12] -> Mux4/2
  [U13] -> Mux4/3
  [U14] -> Mux4/4
  [U16] -> Mux4/6
  [U18] -> Mux4/8
  [U17] -> Mux4/7
  [U22] -> Mux5/2
  [U23] -> Mux5/3
  [U24] -> Mux5/4
  [U28] -> Mux5/8
  [U27] -> Mux5/7
  [U26] -> Mux5/6
  [U32] -> Mux6/2
  [U33] -> Mux6/3
  [U34] -> Mux6/4
  [U38] -> Mux6/8
  [U37] -> Mux6/7
  [U36] -> Mux6/6
  [U42] -> Mux7/2
  [U43] -> Mux7/3
  [U44] -> Mux7/4
  [U48] -> Mux7/8
  [U47] -> Mux7/7
  [U46] -> Mux7/6
  Mux8/1 -> I1/1
  Mux9/1 -> U1/1
  Mux10/1 -> Id/1
  Constant/1 -> Interrupteur/1
  Amp1/1 -> [Id1]
  Constant1/1 -> Interrupteur1/1
  Amp2/1 -> [Id2]
  Constant2/1 -> Interrupteur2/1
  Amp3/1 -> [Id3]
  Constant3/1 -> Interrupteur3/1
  Amp4/1 -> [Id4]
  [Id1] -> Mux10/1
  [Id2] -> Mux10/2
  [Id3] -> Mux10/3
  [Id4] -> Mux10/4
  connections:
  Cellule 2.1/RConn2 -- Cellule 2.2/RConn1
  Cellule 3.8/RConn2 -- Cellule 3.9/RConn1
  Cellule 3.6/RConn2 -- Cellule 3.7/RConn1
  Cellule 4.3/RConn2 -- Cellule 4.4/RConn1
  Cellule 3.4/RConn2 -- Cellule 3.5/RConn1
  Cellule 4.1/RConn2 -- Cellule 4.2/RConn1
  Cellule 3.2/RConn2 -- Cellule 3.3/RConn1
  Cellule 4.2/RConn2 -- Cellule 4.3/RConn1
  Cellule 3.3/RConn2 -- Cellule 3.4/RConn1
  Cellule 3.7/RConn2 -- Cellule 3.8/RConn1
  Cellule 3.5/RConn2 -- Cellule 3.6/RConn1
  Cellule 3.1/RConn2 -- Cellule 3.2/RConn1
  +/RConn1 -- Cellule 1.1/RConn1 -- Shunt 1/RConn1
  Cellule 2.4/RConn2 -- Cellule 2.5/RConn1
  Cellule 2.5/RConn2 -- Cellule 2.6/RConn1
  Cellule 2.2/RConn2 -- Cellule 2.3/RConn1
  Cellule 2.3/RConn2 -- Cellule 2.4/RConn1
  Cellule 2.6/RConn2 -- Cellule 2.7/RConn1
  Cellule 1.1/RConn2 -- Cellule 1.2/RConn1
  Cellule 1.4/RConn2 -- Cellule 1.5/RConn1
  Cellule 1.2/RConn2 -- Cellule 1.3/RConn1
  Cellule 1.6/RConn2 -- Cellule 1.7/RConn1
  Cellule 1.7/RConn2 -- Cellule 1.8/RConn1
  Cellule 1.5/RConn2 -- Cellule 1.6/RConn1
  Cellule 1.8/RConn2 -- Cellule 1.9/RConn1
  Cellule 1.3/RConn2 -- Cellule 1.4/RConn1
  Cellule 2.7/RConn2 -- Cellule 2.8/RConn1
  Cellule 2.8/RConn2 -- Cellule 2.9/RConn1
  Cellule 4.4/RConn2 -- Cellule 4.5/RConn1
  Cellule 4.5/RConn2 -- Cellule 4.6/RConn1
  Cellule 4.6/RConn2 -- Cellule 4.7/RConn1
  Cellule 4.7/RConn2 -- Cellule 4.8/RConn1
  Cellule 4.8/RConn2 -- Cellule 4.9/RConn1
  -/RConn1 -- Cellule 4.9/RConn2 -- Interrupteur3/LConn1
  Cellule 2.1/RConn1 -- Shunt 2/RConn1 -- Interrupteur/LConn1 -- Cellule 1.9/RConn2
  Cellule 2.9/RConn2 -- Shunt 3/RConn1 -- Interrupteur1/LConn1 -- Cellule 3.1/RConn1
  Cellule 3.9/RConn2 -- Shunt 4/RConn1 -- Interrupteur2/LConn1 -- Cellule 4.1/RConn1
  Amp1/RConn1 -- Shunt 1/LConn1
  Amp1/LConn1 -- Interrupteur/RConn1
  Amp2/RConn1 -- Shunt 2/LConn1
  Amp2/LConn1 -- Interrupteur1/RConn1
  Amp3/RConn1 -- Shunt 3/LConn1
  Amp3/LConn1 -- Interrupteur2/RConn1
  Amp4/RConn1 -- Shunt 4/LConn1
  Amp4/LConn1 -- Interrupteur3/RConn1

== system Library_SII_2018/Electronique/Photorésistance ==
  E : Inport
  Add : Sum
  Constant : Constant  Value=a
  Constant1 : Constant  Value=b
  Math Function : Math  Operator=10^u  SaturateOnIntegerOverflow=on
  Math Function1 : Math  Operator=log10  SaturateOnIntegerOverflow=on
  Product : Product
  Simulink-PS Converter : nesl_utility/Simulink-PS Converter  PhysicalDomain=network_engine_domain  SubClassName=ps_input  LeftPortType=input  RightPortType=output  PseudoPeriodic=off  Frequencies=[]  NoiseDistribution=none  NoiseParameters=[]  Unit=1  AffineConversion=off  FilteringAndDerivatives=provide  SimscapeFilterOrder=1  InputFilterTimeConstant=0.001  UdotUserProvided=0
  Variable Resistor : fl_lib/Electrical/Electrical Elements/Variable Resistor  Rmin=0 Ohm  i_specify=off  i_priority=None  i=0 A  i_nominal_specify=off  i_nominal_unit=A  i_nominal_value=1  v_specify=off  v_priority=None  v=0 V  v_nominal_specify=off  v_nominal_unit=V  v_nominal_value=1
  2 : PMIOPort  Side=Right
  1 : PMIOPort  Port=2  Side=Left
  R : Outport
  wires:
  Product/1 -> Add/2
  E/1 -> Math Function1/1
  Math Function1/1 -> Product/2
  Constant1/1 -> Add/1
  Constant/1 -> Product/1
  Add/1 -> Math Function/1
  Math Function/1 -> Simulink-PS Converter/1, R/1
  connections:
  Variable Resistor/LConn2 -- 1/RConn1
  Variable Resistor/RConn1 -- 2/RConn1
  Simulink-PS Converter/RConn1 -- Variable Resistor/LConn1

== system Library_SII_2018/Electronique/Puissance-mètre ==
  Bus Creator : BusCreator  Inputs=3
  Current Sensor : fl_lib/Electrical/Electrical Sensors/Current Sensor
  PS-Simulink Converter1 : nesl_utility/PS-Simulink Converter  PhysicalDomain=network_engine_domain  SubClassName=ps_output  LeftPortType=input  RightPortType=output  PseudoPeriodic=off  Frequencies=[]  Unit=1  AffineConversion=off
  Product : Product
  S-PS : nesl_utility/PS-Simulink Converter  PhysicalDomain=network_engine_domain  SubClassName=ps_output  LeftPortType=input  RightPortType=output  PseudoPeriodic=off  Frequencies=[]  Unit=A  AffineConversion=off
  Voltage Sensor : fl_lib/Electrical/Electrical Sensors/Voltage Sensor
  E+ : PMIOPort  Side=Left
  S+ : PMIOPort  Port=2  Side=Right
  E- : PMIOPort  Port=3  Side=Left
  P : Outport
  wires:
  S-PS/1 -> Bus Creator/2, Product/1  "I"
  PS-Simulink Converter1/1 -> Bus Creator/1, Product/2  "U"
  Product/1 -> Bus Creator/3  "P"
  Bus Creator/1 -> P/1
  connections:
  Current Sensor/RConn1 -- S-PS/LConn1
  Current Sensor/LConn1 -- E+/RConn1 -- Voltage Sensor/LConn1
  S+/RConn1 -- Current Sensor/RConn2
  E-/RConn1 -- Voltage Sensor/RConn2
  Voltage Sensor/RConn1 -- PS-Simulink Converter1/LConn1

== system Library_SII_2018/Electronique/Simscape<->SPS ==
  Controlled Current Source : powerlib/Electrical Sources/Controlled Current Source  Initialize=on  Source_Type=AC  Amplitude=0  Phase=0  Frequency=0  Measurements=None
      settings: SourceProductName=Simscape Electrical
  Controlled Voltage Source : fl_lib/Electrical/Electrical Sources/Controlled Voltage Source
  Current Sensor : fl_lib/Electrical/Electrical Sensors/Current Sensor
  PS-S I : nesl_utility/PS-Simulink Converter  PhysicalDomain=network_engine_domain  SubClassName=ps_output  LeftPortType=input  RightPortType=output  PseudoPeriodic=off  Frequencies=[]  Unit=1  AffineConversion=off
  S-PS V : nesl_utility/Simulink-PS Converter  PhysicalDomain=network_engine_domain  SubClassName=ps_input  LeftPortType=input  RightPortType=output  PseudoPeriodic=off  Frequencies=[]  NoiseDistribution=none  NoiseParameters=[]  Unit=1  AffineConversion=off  FilteringAndDerivatives=zero  SimscapeFilterOrder=1  InputFilterTimeConstant=.001  UdotUserProvided=0
  Series RLC Branch : powerlib/Elements/Series RLC Branch  LConnTagsString=__new0  RConnTagsString=__new0  BranchType=R  Resistance=1e12  Inductance=1e-3  SetiL0=off  InitialCurrent=0  Capacitance=1e-6  Setx0=off  InitialVoltage=0  Measurements=None
      settings: SourceProductName=Simscape Electrical
  Voltage Measurement : powerlib/Measurements/Voltage Measurement  PhasorSimulation=off  OutputType=Complex  PSBequivalent=0
      settings: SourceProductName=Simscape Electrical
  SPS + : PMIOPort  Side=Right
  SS + : PMIOPort  Port=2  Side=Left
  SPS - : PMIOPort  Port=3  Side=Right
  SS - : PMIOPort  Port=4  Side=Left
  wires:
  PS-S I/1 -> Controlled Current Source/1
  Voltage Measurement/1 -> S-PS V/1
  connections:
  SS -/RConn1 -- Controlled Voltage Source/RConn2
  SPS -/RConn1 -- Voltage Measurement/LConn2
  SS +/RConn1 -- Current Sensor/LConn1
  Series RLC Branch/RConn1 -- Controlled Current Source/RConn1 -- SPS +/RConn1
  PS-S I/LConn1 -- Current Sensor/RConn1
  S-PS V/RConn1 -- Controlled Voltage Source/RConn1
  Current Sensor/RConn2 -- Controlled Voltage Source/LConn1
  Series RLC Branch/LConn1 -- Controlled Current Source/LConn1 -- Voltage Measurement/LConn1

== system Library_SII_2018/Electronique/Voltmètre ==
  PS-Simulink Converter1 : nesl_utility/PS-Simulink Converter  PhysicalDomain=network_engine_domain  SubClassName=ps_output  LeftPortType=input  RightPortType=output  PseudoPeriodic=off  Frequencies=[]  Unit=1  AffineConversion=off
  Voltage Sensor : fl_lib/Electrical/Electrical Sensors/Voltage Sensor
  Conn1 : PMIOPort  Side=Left
  Conn2 : PMIOPort  Port=2  Side=Right
  Out1 : Outport
  wires:
  PS-Simulink Converter1/1 -> Out1/1
  connections:
  Voltage Sensor/RConn1 -- PS-Simulink Converter1/LConn1
  Conn1/RConn1 -- Voltage Sensor/LConn1
  Conn2/RConn1 -- Voltage Sensor/RConn2

== system Library_SII_2018/Mécanique/Capteur de force FSR ==
  E : Inport
  Add : Sum
  Constant : Constant  Value=a
  Constant1 : Constant  Value=b
  Math Function : Math  Operator=10^u  SaturateOnIntegerOverflow=on
  Math Function1 : Math  Operator=log10  SaturateOnIntegerOverflow=on
  Product : Product
  Simulink-PS Converter : nesl_utility/Simulink-PS Converter  PhysicalDomain=network_engine_domain  SubClassName=ps_input  LeftPortType=input  RightPortType=output  PseudoPeriodic=off  Frequencies=[]  NoiseDistribution=none  NoiseParameters=[]  Unit=1  AffineConversion=off  FilteringAndDerivatives=provide  SimscapeFilterOrder=1  InputFilterTimeConstant=0.001  UdotUserProvided=0
  Variable Resistor : fl_lib/Electrical/Electrical Elements/Variable Resistor  Rmin=0 Ohm  i_specify=off  i_priority=None  i=0 A  i_nominal_specify=off  i_nominal_unit=A  i_nominal_value=1  v_specify=off  v_priority=None  v=0 V  v_nominal_specify=off  v_nominal_unit=V  v_nominal_value=1
  2 : PMIOPort  Side=Right
  1 : PMIOPort  Port=2  Side=Left
  R : Outport
  wires:
  Product/1 -> Add/2
  E/1 -> Math Function1/1
  Math Function1/1 -> Product/2
  Constant1/1 -> Add/1
  Constant/1 -> Product/1
  Add/1 -> Math Function/1
  Math Function/1 -> Simulink-PS Converter/1, R/1
  connections:
  Variable Resistor/LConn2 -- 1/RConn1
  Variable Resistor/RConn1 -- 2/RConn1
  Simulink-PS Converter/RConn1 -- Variable Resistor/LConn1

== system Library_SII_2018/Mécanique/Capteur de puissance mécanique de rotation ==
  Ideal Rotational Motion Sensor : fl_lib/Mechanical/Mechanical Sensors/Ideal Rotational Motion Sensor  offset=0 rad
  Ideal Torque Sensor : fl_lib/Mechanical/Mechanical Sensors/Ideal Torque Sensor
  PS-Simulink Converter : nesl_utility/PS-Simulink Converter  PhysicalDomain=network_engine_domain  SubClassName=ps_output  LeftPortType=input  RightPortType=output  PseudoPeriodic=off  Frequencies=[]  Unit=1  AffineConversion=off
  PS-Simulink Converter1 : nesl_utility/PS-Simulink Converter  PhysicalDomain=network_engine_domain  SubClassName=ps_output  LeftPortType=input  RightPortType=output  PseudoPeriodic=off  Frequencies=[]  Unit=1  AffineConversion=off
  Product : Product  RndMeth=Zero
  Ref : PMIOPort  Tag=PMCPort  Side=Left
  E : PMIOPort  Port=2  Side=Left
  S : PMIOPort  Tag=PMCPort  Port=3  Side=Right
  P : Outport
  C : Outport  Port=2
  W : Outport  Port=3
  wires:
  PS-Simulink Converter/1 -> C/1, Product/1
  PS-Simulink Converter1/1 -> W/1, Product/2
  Product/1 -> P/1
  connections:
  Ideal Torque Sensor/LConn1 -- E/RConn1
  Ideal Torque Sensor/RConn1 -- S/RConn1 -- Ideal Rotational Motion Sensor/RConn1
  Ideal Rotational Motion Sensor/LConn1 -- Ref/RConn1
  Ideal Rotational Motion Sensor/RConn2 -- PS-Simulink Converter1/LConn1
  Ideal Torque Sensor/RConn2 -- PS-Simulink Converter/LConn1

== system Library_SII_2018/Mécanique/Codeur incrémental ==
  Ideal Rotational Motion Sensor : fl_lib/Mechanical/Mechanical Sensors/Ideal Rotational Motion Sensor  offset=0 rad
  PS-Simulink Converter : nesl_utility/PS-Simulink Converter  PhysicalDomain=network_engine_domain  SubClassName=ps_output  LeftPortType=input  RightPortType=output  PseudoPeriodic=off  Frequencies=[]  Unit=1  AffineConversion=off
  Quantizer : Quantizer  QuantizationInterval=p
  conversion en ° : Gain  Gain=180/pi
  A : PMIOPort  Side=Left
  Ref : PMIOPort  Port=2  Side=Left
  a reel [°] : Outport
  a mes [°] : Outport  Port=2
  wires:
  PS-Simulink Converter/1 -> conversion en °/1
  Quantizer/1 -> a mes [°]/1
  conversion en °/1 -> a reel [°]/1, Quantizer/1
  connections:
  PS-Simulink Converter/LConn1 -- Ideal Rotational Motion Sensor/RConn3
  Ref/RConn1 -- Ideal Rotational Motion Sensor/RConn1
  A/RConn1 -- Ideal Rotational Motion Sensor/LConn1

== system Library_SII_2018/Mécanique/Codeur incrémental v2 ==
  Electrical Reference : fl_lib/Electrical/Electrical Elements/Electrical Reference
  Gain : Gain  Gain=180/pi
  Ideal Rotational Motion Sensor : fl_lib/Mechanical/Mechanical Sensors/Ideal Rotational Motion Sensor  offset=0 rad
  Incremental Shaft Encoder : elec_lib/Sensors/Incremental Shaft Encoder  NPulse=360/p  Vm=U V  angle0=0 deg
      settings: SourceProductName=Simscape Electronics  SourceProductBaseCode=SN
  PS-Simulink Converter{1..4} (4 alike) : nesl_utility/PS-Simulink Converter  PhysicalDomain=network_engine_domain  SubClassName=ps_output  LeftPortType=input  RightPortType=output  PseudoPeriodic=off  Frequencies=[]  Unit=1  AffineConversion=off
  Voltage Sensor : fl_lib/Electrical/Electrical Sensors/Voltage Sensor
  Voltage Sensor1 : fl_lib/Electrical/Electrical Sensors/Voltage Sensor
  Voltage Sensor2 : fl_lib/Electrical/Electrical Sensors/Voltage Sensor
  R : PMIOPort  Side=Left
  C : PMIOPort  Port=2  Side=Left
  A : Outport
  B : Outport  Port=2
  Z : Outport  Port=3
  ar : Outport  Port=4
  wires:
  PS-Simulink Converter1/1 -> A/1
  PS-Simulink Converter2/1 -> B/1
  PS-Simulink Converter3/1 -> Z/1
  PS-Simulink Converter4/1 -> Gain/1
  Gain/1 -> ar/1
  connections:
  C/RConn1 -- Ideal Rotational Motion Sensor/RConn1 -- Incremental Shaft Encoder/LConn2
  R/RConn1 -- Ideal Rotational Motion Sensor/LConn1 -- Incremental Shaft Encoder/LConn1
  Voltage Sensor/LConn1 -- Incremental Shaft Encoder/RConn1
  Voltage Sensor1/LConn1 -- Voltage Sensor2/LConn1 -- Incremental Shaft Encoder/RConn2
  Voltage Sensor1/RConn2 -- Incremental Shaft Encoder/RConn4 -- Voltage Sensor/RConn2
  PS-Simulink Converter1/LConn1 -- Voltage Sensor/RConn1
  PS-Simulink Converter2/LConn1 -- Voltage Sensor1/RConn1
  PS-Simulink Converter3/LConn1 -- Voltage Sensor2/RConn1
  Voltage Sensor2/RConn2 -- Electrical Reference/LConn1 -- Incremental Shaft Encoder/RConn3
  PS-Simulink Converter4/LConn1 -- Ideal Rotational Motion Sensor/RConn3

== system Library_SII_2018/Mécanique/Corde ==
  Calcul de la raideur : MATLAB Function  TreatAsAtomicUnit=on
  Ideal Translational Motion Sensor : fl_lib/Mechanical/Mechanical Sensors/Ideal Translational Motion Sensor  offset=0 m
  Longueur corde [m] : Constant  Value=L
  Module de Young [Pa] : Constant  Value=E*1e12
  PS-Simulink Converter3 : nesl_utility/PS-Simulink Converter  PhysicalDomain=network_engine_domain  SubClassName=ps_output  LeftPortType=input  RightPortType=output  PseudoPeriodic=off  Frequencies=[]  Unit=1  AffineConversion=on
  Ressort lineaire (raideur variable) : Simscape_SII_lib/Ressort lineaire (raideur variable)  v_specify=off  v_priority=High  v=0 m/s  v_nominal_specify=off  v_nominal_unit=m/s  v_nominal_value=1  f_specify=off  f_priority=High  f=0 N  f_nominal_specify=off  f_nominal_unit=N  f_nominal_value=1  x_specify=off  x_priority=High  x=0 m  x_nominal_specify=off  x_nominal_unit=m  x_nominal_value=1
  Section corde [m²] : Constant  Value=S*1e-6
  Simulink-PS Converter1 : nesl_utility/Simulink-PS Converter  PhysicalDomain=network_engine_domain  SubClassName=ps_input  LeftPortType=input  RightPortType=output  PseudoPeriodic=off  Frequencies=[]  NoiseDistribution=none  NoiseParameters=[]  Unit=1  AffineConversion=off  FilteringAndDerivatives=filter  SimscapeFilterOrder=1  InputFilterTimeConstant=0.001  UdotUserProvided=1
  R : PMIOPort  Side=Left
  C : PMIOPort  Port=2  Side=Right
  A : Outport
  wires:
  Calcul de la raideur/1(k) -> Simulink-PS Converter1/1
  Section corde [m²]/1 -> Calcul de la raideur/2(S)
  Longueur corde [m]/1 -> Calcul de la raideur/3(L)
  Module de Young [Pa]/1 -> Calcul de la raideur/1(E)
  PS-Simulink Converter3/1 -> A/1
  connections:
  Simulink-PS Converter1/RConn1 -- Ressort lineaire (raideur variable)/LConn2
  C/RConn1 -- Ideal Translational Motion Sensor/RConn1 -- Ressort lineaire (raideur variable)/RConn1
  R/RConn1 -- Ideal Translational Motion Sensor/LConn1 -- Ressort lineaire (raideur variable)/LConn1
  PS-Simulink Converter3/LConn1 -- Ideal Translational Motion Sensor/RConn3

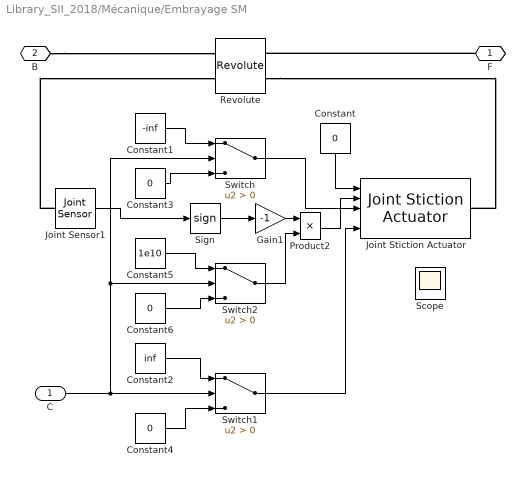
== system Library_SII_2018/Mécanique/Embrayage SM ==
  C : Inport
  Constant{,3..4,6} (4 alike) : Constant  Value=0
  Constant1 : Constant  Value=-inf
  Constant2 : Constant  Value=inf
  Constant5 : Constant  Value=1e10
  Gain1 : Gain  Gain=-1  SaturateOnIntegerOverflow=on  OutDataTypeStr=Inherit: Same as input  ParamDataTypeStr=Inherit: Same as input
  Joint Sensor1 : mblibv1/Sensors &  Actuators/Joint Sensor  UpdateFromCAD=off  PhysicalDomain=Mechanical  PortType=blob  Muxed=off  Pose=off  Angle=off  AngleUnits=deg  ArcVelocity=on  ArcVelocityUnits=rad/s  ArcAcceleration=off  ArcAccelerationUnits=deg/s^2  CoordPosition=on  CoordPositionUnits=m  Velocity=off  VelocityUnits=m/s  Acceleration=off  AccelerationUnits=m/s^2  Quaternion=on  QuaternionDT=off  QuaternionDDT=off  QuaternionUnits=off  OutputVector=[1]  ActiveIO=on  Width=1  DialogClass=MechanicalSensorBlock  Primitive=R1  Force=off  ForceUnits=N  Torque=off  TorqueUnits=N*m  ReferenceFrame=Absolute (World)  ReactionSensedSide=Base  ReactionReferenceFrame=Absolute (World)  ReactionForce=off  ReactionForceUnits=N  ReactionMoment=off  ReactionMomentUnits=N*m
      settings: SourceProductName=Simscape Multibody  SourceProductBaseCode=MS
  Joint Stiction Actuator : mblibv1/Sensors &  Actuators/Joint Stiction Actuator  UpdateFromCAD=off  PhysicalDomain=Mechanical  PortType=blob  ActuationStyle=Force  AngleUnits=deg  ArcVelocityUnits=deg/s  ArcAccelerationUnits=deg/s^2  CoordPositionUnits=m  VelocityUnits=m/s  AccelerationUnits=m/s^2  ForceUnits=N  TorqueUnits=N-m  ActiveIO=on  Width=5  DialogClass=EventActuatorBlock  Primitive=R1  FrictionalForceUnits=N  ExternalForceUnits=N  FrictionalTorqueUnits=N*m  ExternalTorqueUnits=N*m  LockingTolerance=1e-2
      settings: SourceProductName=Simscape Multibody  SourceProductBaseCode=MS
  Product2 : Product  SaturateOnIntegerOverflow=on  InputSameDT=on  OutDataTypeStr=Inherit: Same as first input
  Revolute : mblibv1/Joints/Revolute  LConnTagsString=__newl0|SA1  RConnTagsString=__newr0|SA1  UpdateFromCAD=off  NumSAPorts=2  CutJoint=off  MarkAsCut=off  Primitives=prismatic  PrimitiveProps=R1$World$axe$revolute  DialogClass=JointBlock  R1Axis=axe
      settings: SourceProductName=Simscape Multibody  SourceProductBaseCode=MS
  Scope : Scope
  Sign : Signum  ZeroCross=off
  Switch : Switch  Criteria=u2 > Threshold
  Switch1 : Switch  Criteria=u2 > Threshold
  Switch2 : Switch  Criteria=u2 > Threshold
  F : PMIOPort  Side=Right
  B : PMIOPort  Port=2  Side=Left
  wires:
  Switch2/1 -> Product2/2
  Product2/1 -> Joint Stiction Actuator/2
  Gain1/1 -> Product2/1
  Sign/1 -> Gain1/1
  Joint Sensor1/1 -> Sign/1
  Constant5/1 -> Switch2/1
  Constant6/1 -> Switch2/3
  Constant2/1 -> Switch1/1
  Constant4/1 -> Switch1/3
  Constant1/1 -> Switch/1
  Constant3/1 -> Switch/3
  C/1 -> Switch2/2, Switch/2, Switch1/2
  Switch1/1 -> Joint Stiction Actuator/5
  Switch/1 -> Joint Stiction Actuator/3
  Constant/1 -> Joint Stiction Actuator/1
  connections:
  B/RConn1 -- Revolute/LConn1
  F/RConn1 -- Revolute/RConn1
  Revolute/RConn2 -- Joint Stiction Actuator/RConn1
  Joint Sensor1/LConn1 -- Revolute/LConn2
